simulink model "queue_populator_modeling"  (R2020b)
settings: Solver=FixedStepDiscrete  StartTime=0.0  StopTime=10.0  FixedStep=0.1  RelTol=1e-3
settings Model: Creator=rsub  LastModifiedBy=rsub

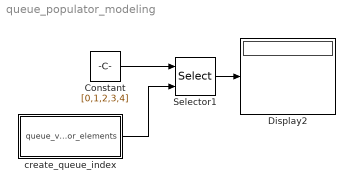
== system queue_populator_modeling ==
  Constant : Constant  Value=[0,1,2,3,4]
  Display2 : Display
  Selector1 : Selector  IndexMode=Zero-based  InputPortWidth=5  IndexOptions=Index vector (port)  Indices=[1 3]  OutputSizes=1
  create_queue_index : Subsystem
  wires:
  create_queue_index/1(queue_vector_elements) -> Selector1/2
  Selector1/1 -> Display2/1
  Constant/1 -> Selector1/1

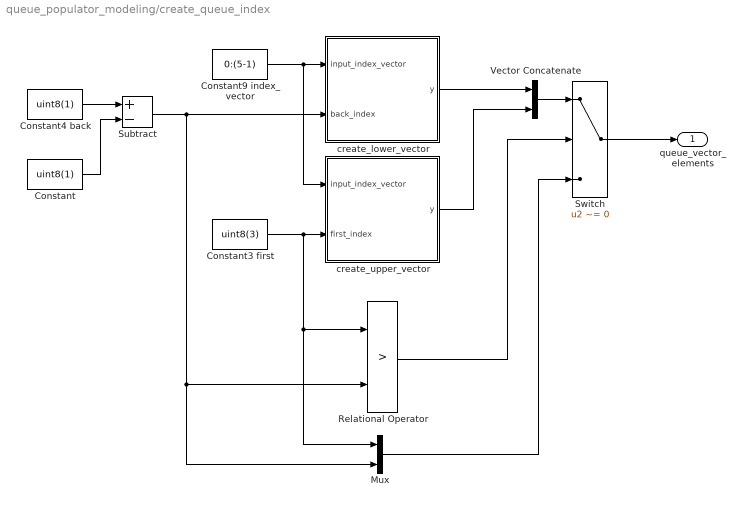
== system queue_populator_modeling/create_queue_index ==
  Constant : Constant  Value=uint8(1)
  Constant3 first : Constant  Value=uint8(3)
  Constant4 back : Constant  Value=uint8(1)
  Constant9 index_vector : Constant  Value=0:(5-1)
  Mux : Mux  Inputs=2
  Relational Operator : RelationalOperator  Operator=>  OutDataTypeStr=boolean  RndMeth=Simplest
  Subtract : Sum  Inputs=+-
  Switch : Switch  Criteria=u2 ~= 0  AllowDiffInputSizes=on
  Vector Concatenate : Concatenate
  create_lower_vector : Subsystem
  create_upper_vector : Subsystem
  queue_vector_elements : Outport
  wires:
  Relational Operator/1 -> Switch/2
  Switch/1 -> queue_vector_elements/1
  Constant9 index_vector/1 -> create_upper_vector/1(input_index_vector), create_lower_vector/1(input_index_vector)
  Vector Concatenate/1 -> Switch/1
  Mux/1 -> Switch/3
  Constant3 first/1 -> Relational Operator/1, Mux/1, create_upper_vector/2(first_index)
  create_upper_vector/1(y) -> Vector Concatenate/2
  create_lower_vector/1(y) -> Vector Concatenate/1
  Subtract/1 -> create_lower_vector/2(back_index), Relational Operator/2, Mux/2
  Constant4 back/1 -> Subtract/1
  Constant/1 -> Subtract/2

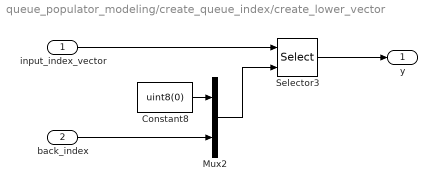
== system queue_populator_modeling/create_queue_index/create_lower_vector ==
  input_index_vector : Inport
  back_index : Inport  Port=2
  Constant8 : Constant  Value=uint8(0)
  Mux2 : Mux  Inputs=2
  Selector3 : Selector  IndexMode=Zero-based  InputPortWidth=5  IndexOptions=Starting and ending indices (port)  Indices=[1 3]  OutputSizes=1
  y : Outport
  wires:
  input_index_vector/1 -> Selector3/1
  Selector3/1 -> y/1
  Constant8/1 -> Mux2/1
  Mux2/1 -> Selector3/2
  back_index/1 -> Mux2/2

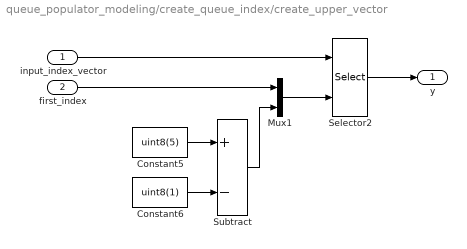
== system queue_populator_modeling/create_queue_index/create_upper_vector ==
  input_index_vector : Inport
  first_index : Inport  Port=2
  Constant5 : Constant  Value=uint8(5)
  Constant6 : Constant  Value=uint8(1)
  Mux1 : Mux  Inputs=2
  Selector2 : Selector  IndexMode=Zero-based  InputPortWidth=5  IndexOptions=Starting and ending indices (port)  Indices=[1 3]  OutputSizes=1
  Subtract : Sum  Inputs=+-
  y : Outport
  wires:
  input_index_vector/1 -> Selector2/1
  Selector2/1 -> y/1
  Constant6/1 -> Subtract/2
  Constant5/1 -> Subtract/1
  first_index/1 -> Mux1/1
  Mux1/1 -> Selector2/2
  Subtract/1 -> Mux1/2
